simulink model "train_dynamic"  (R2018b)
settings: Solver=ode45  StartTime=0.0  StopTime=900  MaxStep=0.001  RelTol=1e-3
settings Model: Creator=LaAir  LastModifiedBy=LaAir

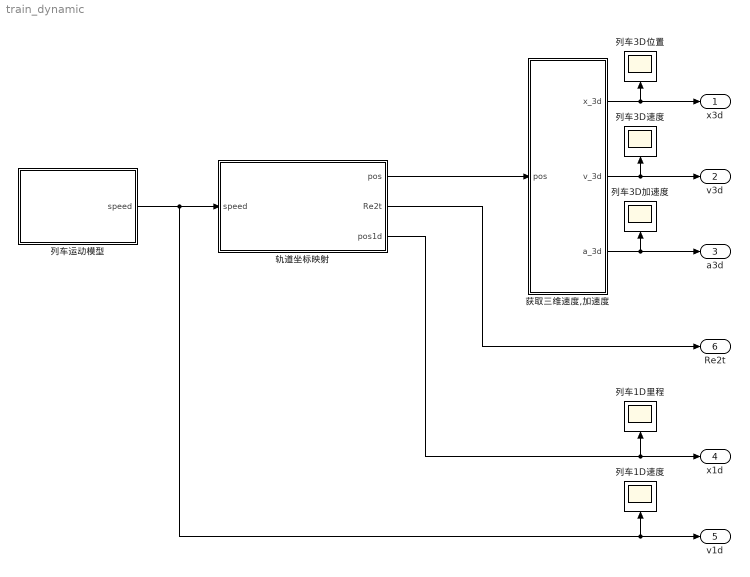
== system train_dynamic ==
  列车1D速度 : Scope
  列车1D里程 : Scope
  列车3D位置 : Scope
  列车3D加速度 : Scope
  列车3D速度 : Scope
  列车运动模型 : Subsystem
  获取三维速度,加速度 : Subsystem
  轨道坐标映射 : Subsystem
  x3d : Outport
  v3d : Outport  Port=2
  a3d : Outport  Port=3
  x1d : Outport  Port=4
  v1d : Outport  Port=5
  Re2t : Outport  Port=6
  wires:
  获取三维速度,加速度/1(x_3d) -> 列车3D位置/1, x3d/1
  获取三维速度,加速度/3(a_3d) -> 列车3D加速度/1, a3d/1
  轨道坐标映射/1(pos) -> 获取三维速度,加速度/1(pos)
  轨道坐标映射/2(Re2t) -> Re2t/1
  轨道坐标映射/3(pos1d) -> x1d/1, 列车1D里程/1
  获取三维速度,加速度/2(v_3d) -> 列车3D速度/1, v3d/1
  列车运动模型/1(speed) -> 轨道坐标映射/1(speed), 列车1D速度/1, v1d/1

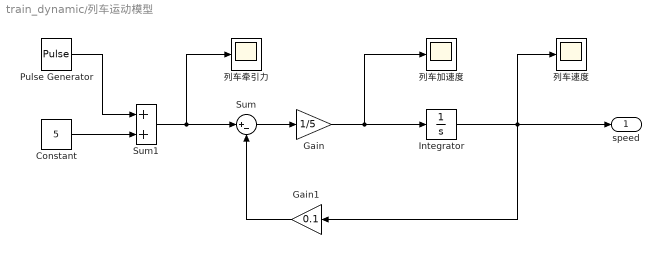
== system train_dynamic/列车运动模型 ==
  Constant : Constant  Value=5
  Gain : Gain  Gain=1/5
  Gain1 : Gain  Gain=0.1
  Integrator : Integrator
  Pulse Generator : DiscretePulseGenerator  PulseType=Time based  Amplitude=5  Period=600  PulseWidth=50
  Sum : Sum  Inputs=|+-
  Sum1 : Sum
  列车加速度 : Scope
  列车牵引力 : Scope
  列车速度 : Scope
  speed : Outport
  wires:
  Gain1/1 -> Sum/2
  Integrator/1 -> 列车速度/1, speed/1, Gain1/1
  Sum/1 -> Gain/1
  Gain/1 -> 列车加速度/1, Integrator/1
  Constant/1 -> Sum1/2
  Pulse Generator/1 -> Sum1/1
  Sum1/1 -> 列车牵引力/1, Sum/1

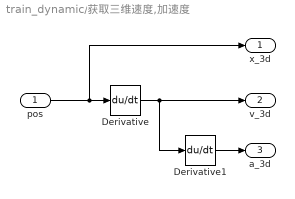
== system train_dynamic/获取三维速度,加速度 ==
  pos : Inport
  Derivative : Derivative
  Derivative1 : Derivative
  x_3d : Outport
  v_3d : Outport  Port=2
  a_3d : Outport  Port=3
  wires:
  Derivative/1 -> v_3d/1, Derivative1/1
  Derivative1/1 -> a_3d/1
  pos/1 -> x_3d/1, Derivative/1

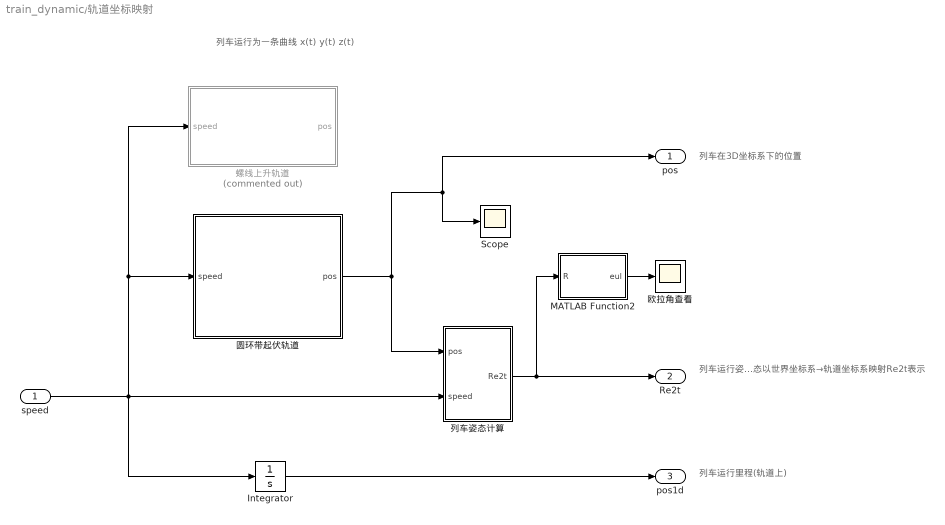
== system train_dynamic/轨道坐标映射 ==
  note: 列车运行为一条曲线
      | x(t) y(t) z(t)
  note: 列车运行里程(轨道上)
  note: 列车在3D坐标系下的位置
  note: 列车运行姿态以世界坐标系→轨道坐标系映射Re2t表示
  speed : Inport
  Integrator : Integrator
  MATLAB Function2 : MATLAB Function  TreatAsAtomicUnit=on
  Scope : Scope
  列车姿态计算 : Subsystem
  圆环带起伏轨道 : Subsystem
  欧拉角查看 : Scope
  螺线上升轨道 : Subsystem  Commented=on
  pos : Outport
  Re2t : Outport  Port=2
  pos1d : Outport  Port=3
  wires:
  speed/1 -> 螺线上升轨道/1(speed), 圆环带起伏轨道/1(speed), 列车姿态计算/2(speed), Integrator/1
  圆环带起伏轨道/1(pos) -> 列车姿态计算/1(pos), Scope/1, pos/1
  Integrator/1 -> pos1d/1
  列车姿态计算/1(Re2t) -> Re2t/1, MATLAB Function2/1(R)
  MATLAB Function2/1(eul) -> 欧拉角查看/1

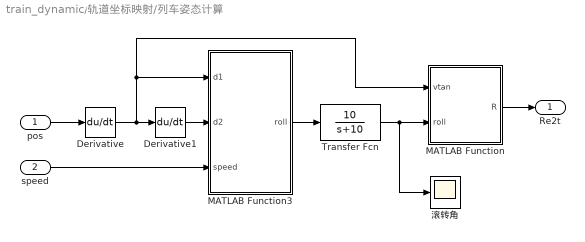
== system train_dynamic/轨道坐标映射/列车姿态计算 ==
  pos : Inport
  speed : Inport  Port=2
  Derivative : Derivative  CoefficientInTFapproximation=100
  Derivative1 : Derivative  CoefficientInTFapproximation=100
  MATLAB Function : MATLAB Function  TreatAsAtomicUnit=on
  MATLAB Function3 : MATLAB Function  TreatAsAtomicUnit=on
  Transfer Fcn : TransferFcn  Numerator=[10]  Denominator=[1 10]
  滚转角 : Scope
  Re2t : Outport
  wires:
  MATLAB Function/1(R) -> Re2t/1
  Derivative1/1 -> MATLAB Function3/2(d2)
  pos/1 -> Derivative/1
  Derivative/1 -> MATLAB Function3/1(d1), MATLAB Function/1(vtan), Derivative1/1
  Transfer Fcn/1 -> 滚转角/1, MATLAB Function/2(roll)
  speed/1 -> MATLAB Function3/3(speed)
  MATLAB Function3/1(roll) -> Transfer Fcn/1

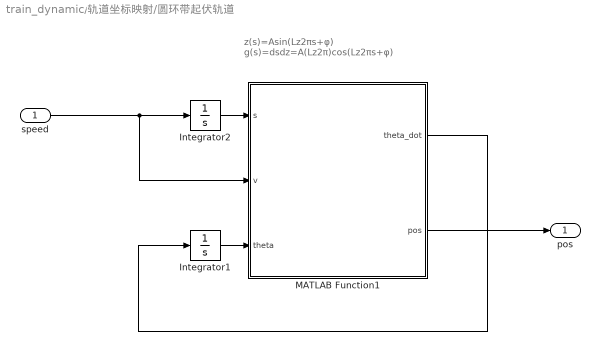
== system train_dynamic/轨道坐标映射/圆环带起伏轨道 ==
  note: z(s)=Asin(Lz​2π​s+φ)
      | g(s)=dsdz​=A(Lz​2π​)cos(Lz​2π​s+φ)
  speed : Inport
  Integrator1 : Integrator
  Integrator2 : Integrator
  MATLAB Function1 : MATLAB Function  TreatAsAtomicUnit=on
  pos : Outport
  wires:
  speed/1 -> MATLAB Function1/2(v), Integrator2/1
  Integrator1/1 -> MATLAB Function1/3(theta)
  Integrator2/1 -> MATLAB Function1/1(s)
  MATLAB Function1/1(theta_dot) -> Integrator1/1
  MATLAB Function1/2(pos) -> pos/1

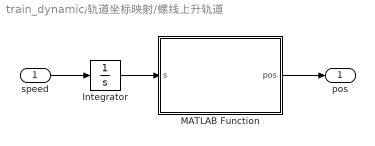
== system train_dynamic/轨道坐标映射/螺线上升轨道 ==
  speed : Inport
  Integrator : Integrator
  MATLAB Function : MATLAB Function  TreatAsAtomicUnit=on
  pos : Outport
  wires:
  MATLAB Function/1(pos) -> pos/1
  Integrator/1 -> MATLAB Function/1(s)
  speed/1 -> Integrator/1

== matlab function train_dynamic/轨道坐标映射/MATLAB Function2 ==
  data: R input; eul output
 function eul = deg(R)
[U, ~, V] = svd(R);
R = U * V';
yaw = atan2(R(2,1),R(1,1));
pitch = asin(-R(3,1));
roll = atan2(R(3,2),R(3,3));
eul = [yaw, pitch, roll]*180/pi;

== matlab function train_dynamic/轨道坐标映射/列车姿态计算/MATLAB Function ==
  data: vtan input; R output; roll input
function R = fcn(vtan, roll)
% --- 轨道姿态 ---
x_axis = vtan / norm(vtan);            % 切向量 = 局部 x 轴
z_world = [0 0 1];           % 世界竖直方向

% Gram–Schmidt 正交化，得到局部 z 轴
z_axis = z_world - dot(z_world, x_axis)*x_axis;
z_axis = z_axis / norm(z_axis);

% y 轴由右手定则确定
y_axis = cross(z_axis, x_axis);
y_axis = y_axis / norm(y_axis);

% 以切向量 x_axis 为旋转轴，绕 roll 旋转
K = [ 0  0  0;
      0  0 -1;
      0  1  0 ];
R_roll = eye(3) + sin(roll)*K + (1-cos(roll))*(K*K);

% 世界->轨道 旋转矩阵 (列向量为局部基)
R = [x_axis(:), y_axis(:), z_axis(:)] * R_roll;

== matlab function train_dynamic/轨道坐标映射/列车姿态计算/MATLAB Function3 ==
  data: d1 input; roll output; d2 input; speed input
function roll = fcn(d1, d2, speed)
r = norm(d1(1:2))^3/norm(d1(1)*d2(2)-d1(2)*d2(1));
g = 9.8;
a = speed^2/r;
a = min(4, a);
roll = atan(a/g);

== matlab function train_dynamic/轨道坐标映射/圆环带起伏轨道/MATLAB Function1 ==
  data: theta_dot output; s input; pos output; v input; theta input
function [theta_dot, pos] = circleUndulate(s, v, theta)
% s    : 弧长（外部由 v 积分得到）
% v    : 速度
% R    : 半径
R = 10000;
% A,Lz,phi: 起伏参数；Lz列车行进多少米完成一次起伏
A = 10; Lz = 10000; phi = 0;
% theta: 当前角
% z0   : 初始高程基准
z0 = 0;
% 输出:
%   theta_dot = dθ/dt (供外部 Integrator)
%   z_dot     = dz/dt (供外部 Integrator, 可选)
%   x,y,z     = 当前位置

omega = 2*pi / Lz;
z_rel = A * sin(omega*s + phi);                % 相对起伏
g = A * omega * cos(omega*s + phi);            % dz/ds
if abs(g) >= 1
    g = 0.999999 * sign(g);
end

omega_s = sqrt(1 - g*g) / R;                   % dθ/ds
theta_dot = omega_s * v;                       % dθ/dt
% z_dot     = g * v;                             % dz/dt (如果想对 z 再积分)
x = R * cos(theta);
y = R * sin(theta);
z = z0 + z_rel;
pos = [x,y,z];
end

== matlab function train_dynamic/轨道坐标映射/螺线上升轨道/MATLAB Function ==
  data: s input; pos output
function pos = mapHelix_byGrade(s)
% s     : 沿轨道弧长（由积分器得到）
% R     : 半径 (m)
R = 10000;
% g     : 坡度 = dz/ds（如 2% 取 0.02）
g = 0.02;
% theta0: 初始角 (rad)
theta0 = 0;
% z0    : 初始高度 (m)
z0 = 0;

% 数值保护，避免 |g|>=1
if abs(g) >= 1
    if g >= 0
        g = 1 - 1e-9;
    else
        g = -1 + 1e-9;
    end
end

omega = sqrt(1 - g*g) / R;      % dθ/ds
theta = theta0 + omega .* s;

x = R .* cos(theta);
y = R .* sin(theta);
z = z0 + g .* s;
pos = [x,y,z];
end
